simulink model "Stabilization_Simulink_Offline_Pendulum_Control"  (R2022b)
settings: Solver=VariableStepAuto  StartTime=0.0  StopTime=30  RelTol=1e-3
undefined symbols (not defined in the file): A, A_ob, B, B_ob, C_full, C_ob, D_full, D_ob, Kpp, voltage_max, x0
settings Model: Creator=utente  LastModifiedBy=federicocorso
settings SolverCC: AlgebraicLoopSolver=TrustRegion
settings DebuggingCC: UnconnectedInputMsg=warning  UnconnectedOutputMsg=warning  UnconnectedLineMsg=warning  SFMachineParentedDataDiag=warning
settings ModelReferenceCC: EnableRefExpFcnMdlSchedulingChecks=on

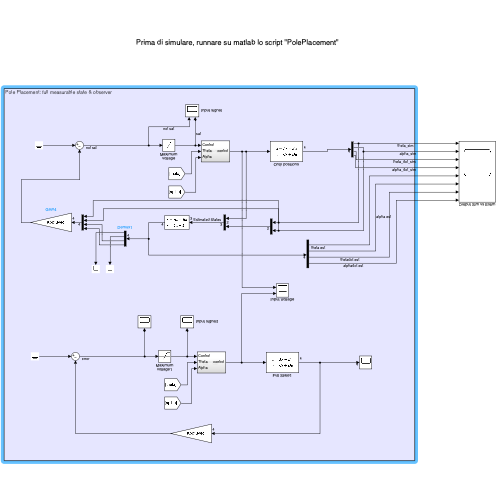
[thumbnail: Simulink's stored preview of the top-level diagram]
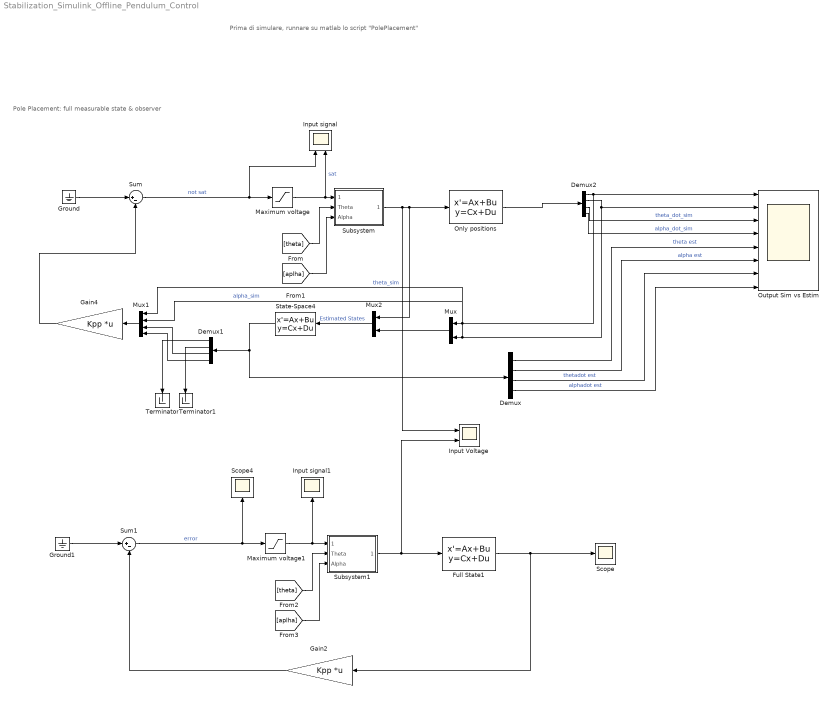
== system Stabilization_Simulink_Offline_Pendulum_Control ==
  note: Pole Placement: full measurable state & observer
  note: Prima di simulare, runnare su matlab lo script "PolePlacement"
  Demux : Demux
  Demux1 : Demux
  Demux2 : Demux
  Full State1 : StateSpace  A=A  B=B  C=C_full  D=D_full  InitialCondition=x0
  Gain2 : Gain  Gain=Kpp  Multiplication=Matrix(K*u) (u vector)
  Gain4 : Gain  Gain=Kpp  Multiplication=Matrix(K*u) (u vector)
  Ground : Ground
  Ground1 : Ground
  Input Voltage : Scope  NumInputPorts=2
  Input signal : Scope  NumInputPorts=2
  Input signal1 : Scope
  Maximum voltage : Saturate  UpperLimit=voltage_max  LowerLimit=-voltage_max
  Maximum voltage1 : Saturate  UpperLimit=voltage_max  LowerLimit=-voltage_max
  Mux : Mux  Inputs=2
  Mux1 : Mux
  Mux2 : Mux  Inputs=2
  Only positions : StateSpace  A=A  B=B  C=C_full  D=D_full  InitialCondition=x0
  Output Sim vs Estim : Scope  NumInputPorts=8
  Scope : Scope
  Scope4 : Scope
  State-Space4 : StateSpace  A=A_ob  B=B_ob  C=C_ob  D=D_ob  InitialCondition=[0;0;0;0]
  Subsystem : Subsystem
  Subsystem1 : Subsystem
  Sum : Sum  Inputs=|+-
  Sum1 : Sum  Inputs=|+-
  Terminator : Terminator
  Terminator1 : Terminator
  wires:
  Maximum voltage/1 -> Input signal/2, Subsystem/1(Control)  "sat"
  [theta] -> Subsystem/2(Theta)
  [aplha] -> Subsystem/3(Alpha)
  Ground/1 -> Sum/1
  Sum/1 -> Input signal/1, Maximum voltage/1  "not sat"
  Gain4/1 -> Sum/2
  Mux2/1 -> State-Space4/1  "Estimated States"
  State-Space4/1 -> Demux1/1, Demux/1
  Subsystem/1(control) -> Mux2/1, Only positions/1, Input Voltage/1
  Sum1/1 -> Maximum voltage1/1, Scope4/1  "error"
  Ground1/1 -> Sum1/1
  Full State1/1 -> Scope/1, Gain2/1
  Subsystem1/1(control) -> Input Voltage/2, Full State1/1
  Maximum voltage1/1 -> Input signal1/1, Subsystem1/1(Control)
  [aplha] -> Subsystem1/3(Alpha)
  [theta] -> Subsystem1/2(Theta)
  Gain2/1 -> Sum1/2
  Demux/1 -> Output Sim vs Estim/5  "theta est"
  Demux/2 -> Output Sim vs Estim/6  "alpha est"
  Demux/3 -> Output Sim vs Estim/7  "thetadot est"
  Demux/4 -> Output Sim vs Estim/8  "alphadot est"
  Only positions/1 -> Demux2/1
  Mux/1 -> Mux2/2
  Demux2/2 -> Output Sim vs Estim/2, Mux1/2, Mux/2  "alpha_sim"
  Demux2/1 -> Output Sim vs Estim/1, Mux1/1, Mux/1  "theta_sim"
  Demux2/3 -> Output Sim vs Estim/3  "theta_dot_sim"
  Demux2/4 -> Output Sim vs Estim/4  "alpha_dot_sim"
  Mux1/1 -> Gain4/1
  Demux1/3 -> Mux1/3
  Demux1/4 -> Mux1/4
  Demux1/1 -> Terminator/1
  Demux1/2 -> Terminator1/1

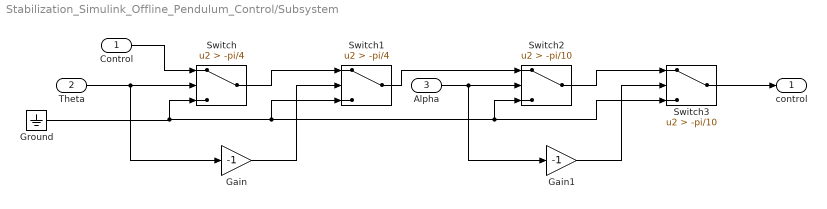
== system Stabilization_Simulink_Offline_Pendulum_Control/Subsystem ==
  Control : Inport
  Theta : Inport  Port=2
  Alpha : Inport  Port=3
  Gain : Gain  Gain=-1
  Gain1 : Gain  Gain=-1
  Ground : Ground
  Switch : Switch  Criteria=u2 > Threshold  Threshold=-pi/4  SaturateOnIntegerOverflow=off  InputSameDT=off
  Switch1 : Switch  Criteria=u2 > Threshold  Threshold=-pi/4  SaturateOnIntegerOverflow=off  InputSameDT=off
  Switch2 : Switch  Criteria=u2 > Threshold  Threshold=-pi/10  SaturateOnIntegerOverflow=off  InputSameDT=off
  Switch3 : Switch  Criteria=u2 > Threshold  Threshold=-pi/10  SaturateOnIntegerOverflow=off  InputSameDT=off
  control : Outport
  wires:
  Gain/1 -> Switch1/2
  Theta/1 -> Gain/1, Switch/2
  Control/1 -> Switch/1
  Switch/1 -> Switch1/1
  Gain1/1 -> Switch3/2
  Switch1/1 -> Switch2/1
  Ground/1 -> Switch3/3, Switch2/3, Switch1/3, Switch/3
  Switch2/1 -> Switch3/1
  Alpha/1 -> Switch2/2, Gain1/1
  Switch3/1 -> control/1

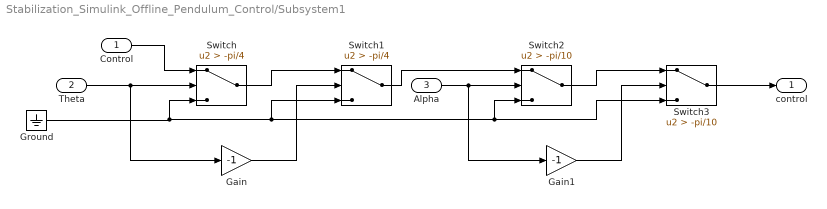
== system Stabilization_Simulink_Offline_Pendulum_Control/Subsystem1 ==
  Control : Inport
  Theta : Inport  Port=2
  Alpha : Inport  Port=3
  Gain : Gain  Gain=-1
  Gain1 : Gain  Gain=-1
  Ground : Ground
  Switch : Switch  Criteria=u2 > Threshold  Threshold=-pi/4  SaturateOnIntegerOverflow=off  InputSameDT=off
  Switch1 : Switch  Criteria=u2 > Threshold  Threshold=-pi/4  SaturateOnIntegerOverflow=off  InputSameDT=off
  Switch2 : Switch  Criteria=u2 > Threshold  Threshold=-pi/10  SaturateOnIntegerOverflow=off  InputSameDT=off
  Switch3 : Switch  Criteria=u2 > Threshold  Threshold=-pi/10  SaturateOnIntegerOverflow=off  InputSameDT=off
  control : Outport
  wires:
  Gain/1 -> Switch1/2
  Theta/1 -> Gain/1, Switch/2
  Control/1 -> Switch/1
  Switch/1 -> Switch1/1
  Gain1/1 -> Switch3/2
  Switch1/1 -> Switch2/1
  Ground/1 -> Switch3/3, Switch2/3, Switch1/3, Switch/3
  Switch2/1 -> Switch3/1
  Alpha/1 -> Switch2/2, Gain1/1
  Switch3/1 -> control/1
